simulink model "one_third"  (R2019a)
settings: Solver=ode4  StartTime=0.0  StopTime=Tf  FixedStep=0.001  RelTol=1e-3
values from neighbouring files (symbols this model uses):
  HzBPF = c2d(HsBPF,Ts,opt1)    [one_discussion_code.m]
  HzBSF = c2d(HsBSF,Ts,opt2)    [one_discussion_code.m]
  HzHPF1 = c2d(HsHPF1,Ts,'tustin')    [one_discussion_code.m]
  HzHPF2 = c2d(HsHPF2,Ts,'tustin')    [one_discussion_code.m]
  HzLPF1 = c2d(HsLPF1,Ts,'tustin')    [one_discussion_code.m]
  HzLPF2 = c2d(HsLPF2,Ts,'tustin')    [one_discussion_code.m]
  Ts = 0.001    [one_discussion_code.m]
  white_noise = sigma^2*Ts    (= 4e-05)    [one_discussion_code.m]
undefined symbols (not defined in the file or in its folder): CT_BPF_DEN, CT_BPF_NUM, CT_BSF_DEN, CT_BSF_NUM, CT_HPF_DEN1, CT_HPF_DEN2, CT_HPF_NUM1, CT_HPF_NUM2, CT_LPF_DEN1, CT_LPF_DEN2, CT_LPF_NUM1, CT_LPF_NUM2
libraries: simulink x2, dspsigops x2
settings Model: Creator=문선빈  LastModifiedBy=문선빈

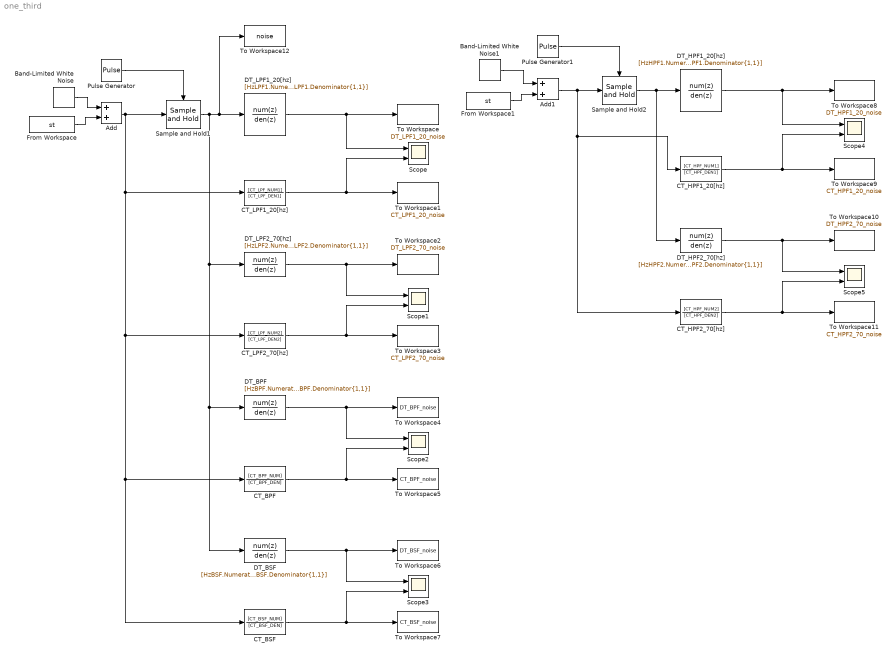
== system one_third ==
  Add : Sum
  Add1 : Sum
  Band-Limited White Noise : simulink/Sources/Band-Limited White Noise  Cov=[white_noise]  Ts=Ts  seed=[23341]
  Band-Limited White Noise1 : simulink/Sources/Band-Limited White Noise  Cov=[white_noise]  Ts=Ts  seed=[23341]
  "CT_BPF " : TransferFcn  Numerator=[CT_BPF_NUM]  Denominator=[CT_BPF_DEN]
  CT_BSF : TransferFcn  Numerator=[CT_BSF_NUM]  Denominator=[CT_BSF_DEN]
  CT_HPF1_20[hz] : TransferFcn  Numerator=[CT_HPF_NUM1]  Denominator=[CT_HPF_DEN1]
  CT_HPF2_70[hz] : TransferFcn  Numerator=[CT_HPF_NUM2]  Denominator=[CT_HPF_DEN2]
  CT_LPF1_20[hz] : TransferFcn  Numerator=[CT_LPF_NUM1]  Denominator=[CT_LPF_DEN1]
  CT_LPF2_70[hz] : TransferFcn  Numerator=[CT_LPF_NUM2]  Denominator=[CT_LPF_DEN2]
  DT_BPF : DiscreteTransferFcn  Numerator=[HzBPF.Numerator{1,1}]  Denominator=[HzBPF.Denominator{1,1}]  SampleTime=Ts
  "DT_BSF " : DiscreteTransferFcn  Numerator=[HzBSF.Numerator{1,1}]  Denominator=[HzBSF.Denominator{1,1}]  SampleTime=Ts
  DT_HPF1_20[hz] : DiscreteTransferFcn  Numerator=[HzHPF1.Numerator{1,1}]  Denominator=[HzHPF1.Denominator{1,1}]  SampleTime=Ts
  DT_HPF2_70[hz] : DiscreteTransferFcn  Numerator=[HzHPF2.Numerator{1,1}]  Denominator=[HzHPF2.Denominator{1,1}]  SampleTime=Ts
  "DT_LPF1_20[hz] " : DiscreteTransferFcn  Numerator=[HzLPF1.Numerator{1,1}]  Denominator=[HzLPF1.Denominator{1,1}]  SampleTime=Ts
  DT_LPF2_70[hz] : DiscreteTransferFcn  Numerator=[HzLPF2.Numerator{1,1}]  Denominator=[HzLPF2.Denominator{1,1}]  SampleTime=Ts
  From Workspace : FromWorkspace  VariableName=st  SampleTime=Ts
  From Workspace1 : FromWorkspace  VariableName=st  SampleTime=Ts
  Pulse Generator : DiscretePulseGenerator  PulseType=Time based  Period=2*Ts  PulseWidth=50
  Pulse Generator1 : DiscretePulseGenerator  PulseType=Time based  Period=0.002  PulseWidth=50
  Sample and Hold1 : dspsigops/Sample and Hold  trig=Rising edge  initCond=0  latchinput=off
  Sample and Hold2 : dspsigops/Sample and Hold  trig=Rising edge  initCond=0  latchinput=off
  Scope{,1..5} (6 alike) : Scope  NumInputPorts=2
  To Workspace : ToWorkspace  VariableName=DT_LPF1_20_noise  SampleTime=Ts
      settings: Save2DSignal=2-D array (concatenate along first dimension)
  To Workspace1 : ToWorkspace  VariableName=CT_LPF1_20_noise  SampleTime=Ts
      settings: Save2DSignal=2-D array (concatenate along first dimension)
  To Workspace10 : ToWorkspace  VariableName=DT_HPF2_70_noise  SampleTime=Ts
      settings: Save2DSignal=2-D array (concatenate along first dimension)
  To Workspace11 : ToWorkspace  VariableName=CT_HPF2_70_noise  SampleTime=Ts
      settings: Save2DSignal=2-D array (concatenate along first dimension)
  To Workspace12 : ToWorkspace  VariableName=noise  SampleTime=Ts
      settings: Save2DSignal=2-D array (concatenate along first dimension)
  To Workspace2 : ToWorkspace  VariableName=DT_LPF2_70_noise  SampleTime=Ts
      settings: Save2DSignal=2-D array (concatenate along first dimension)
  To Workspace3 : ToWorkspace  VariableName=CT_LPF2_70_noise  SampleTime=Ts
      settings: Save2DSignal=2-D array (concatenate along first dimension)
  To Workspace4 : ToWorkspace  VariableName=DT_BPF_noise  SampleTime=Ts
      settings: Save2DSignal=2-D array (concatenate along first dimension)
  To Workspace5 : ToWorkspace  VariableName=CT_BPF_noise  SampleTime=Ts
      settings: Save2DSignal=2-D array (concatenate along first dimension)
  To Workspace6 : ToWorkspace  VariableName=DT_BSF_noise  SampleTime=Ts
      settings: Save2DSignal=2-D array (concatenate along first dimension)
  To Workspace7 : ToWorkspace  VariableName=CT_BSF_noise  SampleTime=Ts
      settings: Save2DSignal=2-D array (concatenate along first dimension)
  To Workspace8 : ToWorkspace  VariableName=DT_HPF1_20_noise  SampleTime=Ts
      settings: Save2DSignal=2-D array (concatenate along first dimension)
  To Workspace9 : ToWorkspace  VariableName=CT_HPF1_20_noise  SampleTime=Ts
      settings: Save2DSignal=2-D array (concatenate along first dimension)
  wires:
  DT_BPF/1 -> Scope2/1, To Workspace4/1
  "CT_BPF "/1 -> To Workspace5/1, Scope2/2
  "DT_BSF "/1 -> Scope3/1, To Workspace6/1
  DT_LPF2_70[hz]/1 -> Scope1/1, To Workspace2/1
  CT_LPF1_20[hz]/1 -> Scope/2, To Workspace1/1
  CT_BSF/1 -> To Workspace7/1, Scope3/2
  Sample and Hold1/1 -> "DT_BSF "/1, DT_BPF/1, DT_LPF2_70[hz]/1, To Workspace12/1, "DT_LPF1_20[hz] "/1
  Pulse Generator/1 -> Sample and Hold1/Trigger
  DT_HPF1_20[hz]/1 -> To Workspace8/1, Scope4/1
  CT_HPF1_20[hz]/1 -> Scope4/2, To Workspace9/1
  Add/1 -> Sample and Hold1/1, CT_LPF2_70[hz]/1, "CT_BPF "/1, CT_BSF/1, CT_LPF1_20[hz]/1
  Add1/1 -> CT_HPF2_70[hz]/1, CT_HPF1_20[hz]/1, Sample and Hold2/1
  Sample and Hold2/1 -> DT_HPF2_70[hz]/1, DT_HPF1_20[hz]/1
  CT_LPF2_70[hz]/1 -> To Workspace3/1, Scope1/2
  "DT_LPF1_20[hz] "/1 -> To Workspace/1, Scope/1
  Pulse Generator1/1 -> Sample and Hold2/Trigger
  CT_HPF2_70[hz]/1 -> To Workspace11/1, Scope5/2
  DT_HPF2_70[hz]/1 -> Scope5/1, To Workspace10/1
  Band-Limited White Noise/1 -> Add/1
  From Workspace/1 -> Add/2
  Band-Limited White Noise1/1 -> Add1/1
  From Workspace1/1 -> Add1/2
